simulink model "bdot_simple_sim"  (R2016b)
settings: Solver=VariableStepAuto  StartTime=0.0  StopTime=10000  RelTol=1e-3  EnableMultiTasking=on
values from neighbouring files (symbols this model uses):
  fsw_params = init_fsw_params()    [bdot_controller_edit_test.m]    (also in bdot_controlller_unit_test.m; bdot_monte_carlo.m)
  sim_params = init_sim_params(fsw_params)    [bdot_controller_edit_test.m]    (also in bdot_controlller_unit_test.m)
undefined symbols (not defined in the file or in its folder): DiscIntNeverNeededParam
libraries: aerolibutil x6, dynamics_lib x2, vrlib x1, GPS_time_lib x1, MSP_BDOT_lib x1, aerolibtransform2 x1, simulink x1, mag_vec_LS_lib x1, magnetometer_lib x1, magnetorquer_assembly_lib x1, sgp4_lib_fsw x1, solar_panel_power_lib x1
settings Model: Creator=Taylor  LastModifiedBy=scrice
settings OptimizationCC: DefaultParameterBehavior=Inlined  UseDivisionForNetSlopeComputation=on  UseFloatMulNetSlope=on  InlineInvariantSignals=on  PassReuseOutputArgsAs=Individual arguments  ZeroExternalMemoryAtStartup=off  ZeroInternalMemoryAtStartup=off  NoFixptDivByZeroProtection=on  EfficientFloat2IntCast=on  LifeSpan=1
settings DebuggingCC: ParameterTunabilityLossMsg=error  SFUnexpectedBacktrackingDiag=warning  SFNoUnconditionalDefaultTransitionDiag=warning  SFExecutionAtInitializationDiag=none
settings HardwareCC: ProdBitPerInt=16  ProdBitPerPointer=16  ProdBitPerSizeT=16  ProdBitPerPtrDiffT=16  ProdLargestAtomicFloat=None  ProdWordSize=16  ProdHWDeviceType=Texas Instruments->MSP430
settings RTWCC: SystemTargetFile=ert.tlc  TemplateMakefile=ert_default_tmf  Description=Embedded Coder  GenerateReport=on  IncludeHyperlinkInReport=on  LaunchReport=on  GenerateTraceInfo=on  GenerateTraceReport=on  GenerateTraceReportSl=on  GenerateTraceReportSf=on  GenerateTraceReportEml=on  GenerateCodeMetricsReport=on
settings CodeAppCC: ForceParamTrailComments=on  IgnoreCustomStorageClasses=off  OperatorAnnotations=on  SimulinkDataObjDesc=on  SFDataObjDesc=on  MATLABFcnDesc=on  CustomSymbolStrGlobalVar=rt$N$M  CustomSymbolStrType=$N$M  CustomSymbolStrFcn=$N$M$F  CustomSymbolStrMacro=$N$M  InsertBlockDesc=on  MATLABSourceComments=on
settings ERTTargetCC: GenerateSampleERTMain=on  CombineSignalStateStructs=on  SupportComplex=off  SupportContinuousTime=on  SupportNonInlinedSFcns=on  InlinedParameterPlacement=NonHierarchical  ERTCustomFileTemplate=example_file_process.tlc  ERTFilePackagingFormat=CompactWithDataFile
settings ConfigComp: CovMetricSettings=dw  CovHtmlReporting=on  CovSaveCumulativeToWorkspaceVar=on  CovSaveSingleToWorkspaceVar=on  CovExternalEMLEnable=off

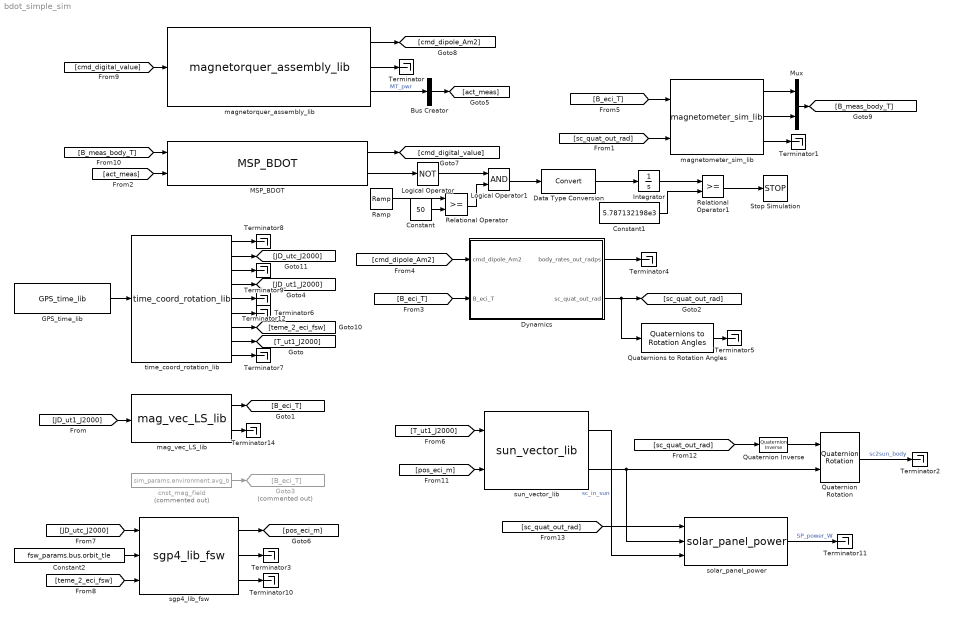
== system bdot_simple_sim ==
  Bus Creator : BusCreator  Inputs=1
  Constant : Constant  Value=50
  Constant1 : Constant  Value=5.787132198e3
  Constant2 : Constant  Value=fsw_params.bus.orbit_tle
  Data Type Conversion : DataTypeConversion
  Dynamics : Subsystem
  GPS_time_lib : GPS_time_lib/GPS_time_lib
  Goto3 : Goto  Commented=on  GotoTag=B_eci_T
  Integrator : Integrator
  Logical Operator : Logic  Operator=NOT  AllPortsSameDT=off  OutDataTypeStr=boolean
  Logical Operator1 : Logic  AllPortsSameDT=off  OutDataTypeStr=boolean
  MSP_BDOT : MSP_BDOT_lib/MSP_BDOT
  Mux : Mux  Inputs=[3 1]
  Quaternion Inverse : aerolibutil/Quaternion Inverse
  Quaternion Rotation : aerolibutil/Quaternion Rotation
  Quaternions to Rotation Angles : aerolibtransform2/Quaternions to Rotation Angles  rotationOrder=XYZ
  Ramp : simulink/Sources/Ramp  slope=1  start=0  X0=0
  Relational Operator : RelationalOperator  OutDataTypeStr=boolean  RndMeth=Simplest
  Relational Operator1 : RelationalOperator  OutDataTypeStr=boolean  RndMeth=Simplest
  Stop Simulation : Stop
  Terminator{,1..12,14} (14 alike) : Terminator
  cnst_mag_field : Constant  Commented=on  Value=sim_params.environment.avg_b
  mag_vec_LS_lib : mag_vec_LS_lib/mag_vec_LS_lib
  magnetometer_sim_lib : magnetometer_lib/magnetometer_sim_lib  seed_x=4  seed_y=5  seed_z=6
  magnetorquer_assembly_lib : magnetorquer_assembly_lib/magnetorquer_assembly_lib
  sgp4_lib_fsw : sgp4_lib_fsw/sgp4_lib_fsw
  solar_panel_power : solar_panel_power_lib/solar_panel_power
  sun_vector_lib : sun_vector_lib/sun_vector_lib
  time_coord_rotation_lib : time_coord_rotation_lib/time_coord_rotation_lib
  wires:
  magnetometer_sim_lib/2 -> Mux/2
  magnetometer_sim_lib/1 -> Mux/1
  magnetometer_sim_lib/3 -> Terminator1/1
  [sc_quat_out_rad] -> magnetometer_sim_lib/2
  Dynamics/1(body_rates_out_radps) -> Terminator4/1
  Dynamics/2(sc_quat_out_rad) -> Quaternions to Rotation Angles/1, [sc_quat_out_rad]
  [cmd_dipole_Am2] -> Dynamics/1(cmd_dipole_Am2)
  [B_eci_T] -> Dynamics/2(B_eci_T)
  [cmd_digital_value] -> magnetorquer_assembly_lib/1
  magnetorquer_assembly_lib/1 -> [cmd_dipole_Am2]
  magnetorquer_assembly_lib/2 -> Terminator/1
  Quaternions to Rotation Angles/1 -> Terminator5/1
  time_coord_rotation_lib/2 -> [JD_utc_J2000]
  time_coord_rotation_lib/3 -> Terminator9/1
  time_coord_rotation_lib/4 -> [JD_ut1_J2000]
  time_coord_rotation_lib/5 -> Terminator12/1
  time_coord_rotation_lib/6 -> Terminator6/1
  time_coord_rotation_lib/7 -> [teme_2_eci_fsw]
  time_coord_rotation_lib/8 -> [T_ut1_J2000]
  time_coord_rotation_lib/9 -> Terminator7/1
  time_coord_rotation_lib/1 -> Terminator8/1
  [JD_ut1_J2000] -> mag_vec_LS_lib/1
  GPS_time_lib/1 -> time_coord_rotation_lib/1
  mag_vec_LS_lib/1 -> [B_eci_T]
  [B_eci_T] -> magnetometer_sim_lib/1
  mag_vec_LS_lib/2 -> Terminator14/1
  cnst_mag_field/1 -> Goto3/1
  Mux/1 -> [B_meas_body_T]
  [B_meas_body_T] -> MSP_BDOT/1
  magnetorquer_assembly_lib/3 -> Bus Creator/1  "MT_pwr"
  Bus Creator/1 -> [act_meas]
  [act_meas] -> MSP_BDOT/2
  MSP_BDOT/1 -> [cmd_digital_value]
  [T_ut1_J2000] -> sun_vector_lib/1
  sgp4_lib_fsw/3 -> Terminator10/1
  sgp4_lib_fsw/2 -> Terminator3/1
  [teme_2_eci_fsw] -> sgp4_lib_fsw/3
  Constant2/1 -> sgp4_lib_fsw/2
  sgp4_lib_fsw/1 -> [pos_eci_m]
  [JD_utc_J2000] -> sgp4_lib_fsw/1
  [pos_eci_m] -> sun_vector_lib/2
  sun_vector_lib/1 -> solar_panel_power/3  "sc_in_sun"
  sun_vector_lib/2 -> solar_panel_power/2, Quaternion Rotation/2
  MSP_BDOT/2 -> Logical Operator/1
  Logical Operator1/1 -> Data Type Conversion/1
  Logical Operator/1 -> Logical Operator1/1
  Relational Operator/1 -> Logical Operator1/2
  Ramp/1 -> Relational Operator/1
  Constant/1 -> Relational Operator/2
  Quaternion Inverse/1 -> Quaternion Rotation/1
  [sc_quat_out_rad] -> Quaternion Inverse/1
  Quaternion Rotation/1 -> Terminator2/1  "sc2sun_body"
  [sc_quat_out_rad] -> solar_panel_power/1
  solar_panel_power/1 -> Terminator11/1  "SP_power_W"
  Integrator/1 -> Relational Operator1/1
  Relational Operator1/1 -> Stop Simulation/1
  Constant1/1 -> Relational Operator1/2
  Data Type Conversion/1 -> Integrator/1

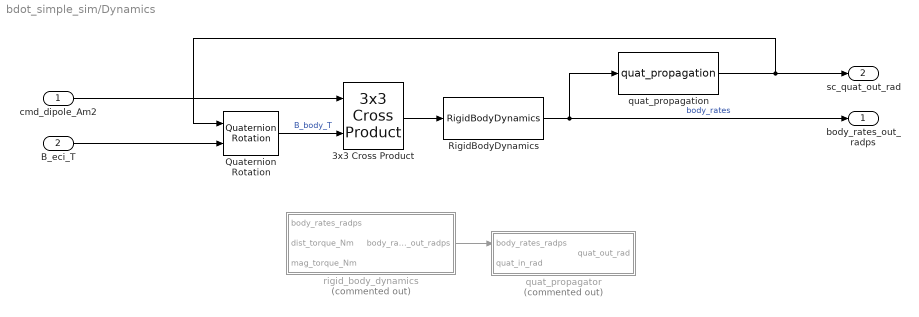
== system bdot_simple_sim/Dynamics ==
  cmd_dipole_Am2 : Inport
  B_eci_T : Inport  Port=2
  3x3 Cross Product : aerolibutil/3x3 Cross Product
  Quaternion Rotation : aerolibutil/Quaternion Rotation
  RigidBodyDynamics : dynamics_lib/Dynamics/RigidBodyDynamics
  quat_propagation : dynamics_lib/Dynamics/quat_propagation
  quat_propagator : Subsystem  Commented=on
  rigid_body_dynamics : Subsystem  Commented=on
  body_rates_out_radps : Outport
  sc_quat_out_rad : Outport  Port=2
  wires:
  Quaternion Rotation/1 -> 3x3 Cross Product/2  "B_body_T"
  cmd_dipole_Am2/1 -> 3x3 Cross Product/1
  rigid_body_dynamics/1(body_rates_out_radps) -> quat_propagator/1(body_rates_radps)
  B_eci_T/1 -> Quaternion Rotation/2
  3x3 Cross Product/1 -> RigidBodyDynamics/1
  RigidBodyDynamics/1 -> body_rates_out_radps/1, quat_propagation/1  "body_rates"
  quat_propagation/1 -> sc_quat_out_rad/1, Quaternion Rotation/1

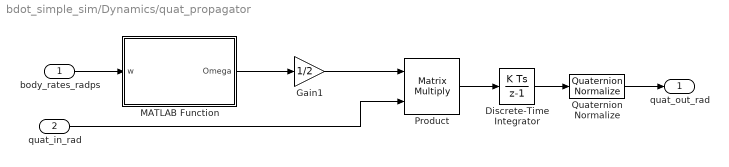
== system bdot_simple_sim/Dynamics/quat_propagator ==
  body_rates_radps : Inport
  quat_in_rad : Inport  Port=2
  Discrete-Time Integrator : DiscreteIntegrator  InitialCondition=sim_params.dynamics.ic.quat_init  InitialConditionSetting=State (most efficient)  SampleTime=fsw_params.sample_time_s  ICPrevOutput=DiscIntNeverNeededParam  ICPrevScaledInput=DiscIntNeverNeededParam
  Gain1 : Gain  Gain=1/2
  MATLAB Function : MATLAB Function  TreatAsAtomicUnit=on
  Product : Product  Multiplication=Matrix(*)  RndMeth=Zero
  Quaternion Normalize : aerolibutil/Quaternion Normalize
  quat_out_rad : Outport
  wires:
  Product/1 -> Discrete-Time Integrator/1
  Quaternion Normalize/1 -> quat_out_rad/1
  Discrete-Time Integrator/1 -> Quaternion Normalize/1
  Gain1/1 -> Product/1
  quat_in_rad/1 -> Product/2
  body_rates_radps/1 -> MATLAB Function/1(w)
  MATLAB Function/1(Omega) -> Gain1/1

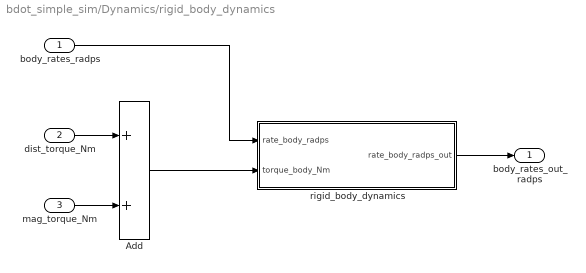
== system bdot_simple_sim/Dynamics/rigid_body_dynamics ==
  body_rates_radps : Inport
  dist_torque_Nm : Inport  Port=2
  mag_torque_Nm : Inport  Port=3
  Add : Sum
  rigid_body_dynamics : Subsystem
  body_rates_out_radps : Outport
  wires:
  dist_torque_Nm/1 -> Add/1
  Add/1 -> rigid_body_dynamics/2(torque_body_Nm)
  mag_torque_Nm/1 -> Add/2
  rigid_body_dynamics/1(rate_body_radps_out) -> body_rates_out_radps/1
  body_rates_radps/1 -> rigid_body_dynamics/1(rate_body_radps)

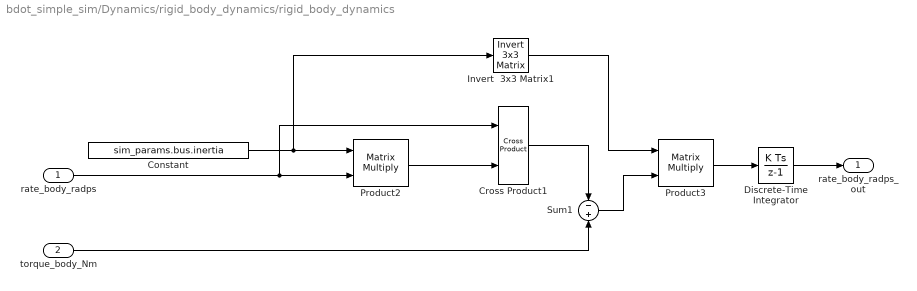
== system bdot_simple_sim/Dynamics/rigid_body_dynamics/rigid_body_dynamics ==
  rate_body_radps : Inport
  torque_body_Nm : Inport  Port=2
  Constant : Constant  Value=sim_params.bus.inertia
  Cross Product1 : vrlib/Utilities/Cross Product
  Discrete-Time Integrator : DiscreteIntegrator  InitialCondition=sim_params.dynamics.ic.rate_init  InitialConditionSetting=State (most efficient)  SampleTime=fsw_params.sample_time_s  ICPrevOutput=DiscIntNeverNeededParam  ICPrevScaledInput=DiscIntNeverNeededParam
  Invert  3x3 Matrix1 : aerolibutil/Invert  3x3 Matrix
  Product2 : Product  Multiplication=Matrix(*)  RndMeth=Zero
  Product3 : Product  Multiplication=Matrix(*)  RndMeth=Zero
  Sum1 : Sum  Inputs=-+
  rate_body_radps_out : Outport
  wires:
  Discrete-Time Integrator/1 -> rate_body_radps_out/1
  Product3/1 -> Discrete-Time Integrator/1
  Invert  3x3 Matrix1/1 -> Product3/1
  Sum1/1 -> Product3/2
  torque_body_Nm/1 -> Sum1/2
  Cross Product1/1 -> Sum1/1
  rate_body_radps/1 -> Product2/2, Cross Product1/1
  Product2/1 -> Cross Product1/2
  Constant/1 -> Product2/1, Invert  3x3 Matrix1/1

== matlab function bdot_simple_sim/Dynamics/quat_propagator/MATLAB Function ==
  data: w input; Omega output
function Omega = skew_sym(w)
%#codegen

    w_skew = ...
        [0 w(3) -w(2);
        -w(3) 0 w(1);
        w(2) -w(1) 0];

    Omega = ...
        [0 -w';
        w w_skew];
